simulink model "sampleModel256"  (R2021b)
settings: Solver=VariableStepAuto  StartTime=0.0  StopTime=10.0  RelTol=1e-3
undefined symbols (not defined in the file or in its folder): DiscIntNeverNeededParam
libraries: simulink x12, slpidlib x1
settings Model: Creator=user  LastModifiedBy=user

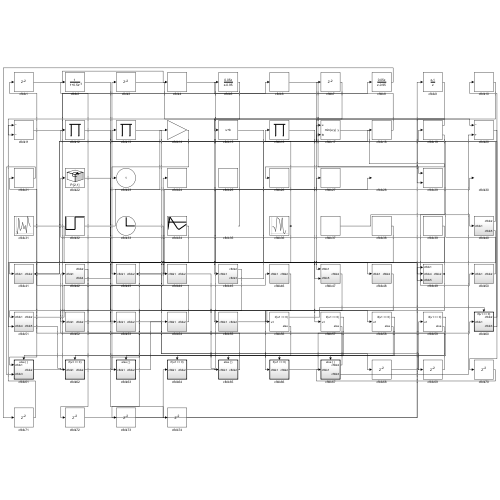
[thumbnail: Simulink's stored preview of the top-level diagram]
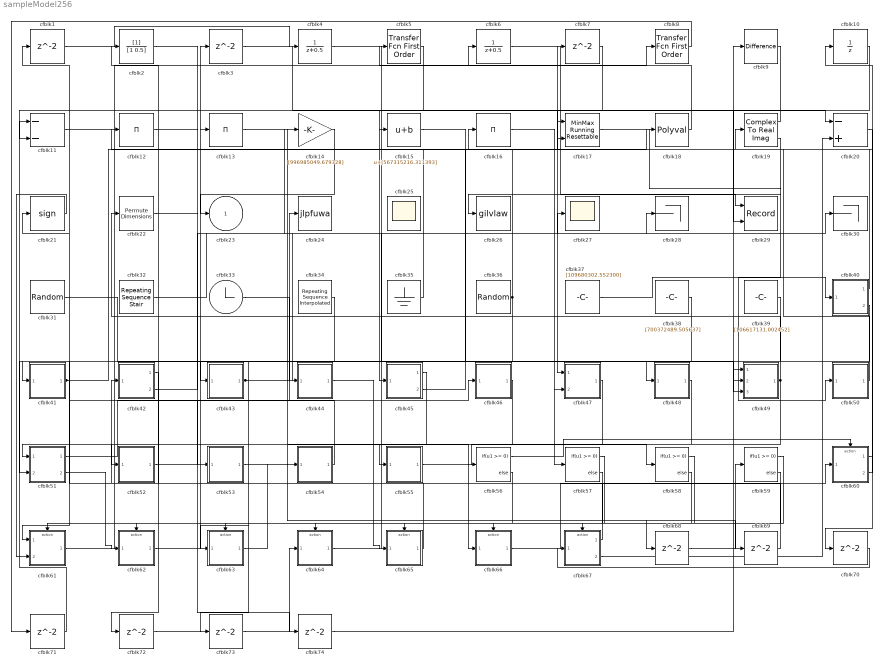
== system sampleModel256 ==
  cfblk{1,3,7,68..74} (10 alike) : Delay  SampleTime=1
  cfblk10 : UnitDelay  HasFrameUpgradeWarning=on
  cfblk11 : Sum  Inputs=--
  cfblk12 : Product  Inputs=*
  cfblk13 : Product  Inputs=*
  cfblk14 : Gain  Gain=[996985049.679328]
  cfblk15 : Bias  Bias=[567315216.311393]
  cfblk16 : Product  Inputs=*
  cfblk17 : simulink/Math Operations/MinMax Running Resettable  Function=min  vinit=0.0
  cfblk18 : Polyval  Coefs=[ +2.081618890e-019, -1.441693666e-014, +4.719686976e-010, -8.536869453e-006, +1.621573104e-001, -8.087801117e+001 ]
  cfblk19 : ComplexToRealImag
  cfblk2 : DiscreteFilter  SampleTime=1
  cfblk20 : Sum  Inputs=-+
  cfblk21 : Signum
  cfblk22 : PermuteDimensions
  cfblk24 : ToWorkspace  VariableName=jlpfuwa  SaveFormat=Timeseries  SampleTime=-1
  cfblk25 : Scope
      settings: Floating=on
  cfblk26 : ToWorkspace  VariableName=gilvlaw  SaveFormat=Timeseries  SampleTime=-1
  cfblk27 : Scope
  cfblk28 : Terminator
  cfblk29 : Record  FileSettingsInternal="{\"entries\":[{\"content\":{\"excelSettings\":{\"content\":{},\"type\":\"Streamout.ExcelSettings\"}},\"type\":\"Streamout.FileSettingStorage\",\"uuid\":\"d0f24451-51db-411e-8607-9f3c8963e8ef\"}],\"packageUris\":[\"http://schema.mathworks.com/mf0/streamout_blocks/R2020a\"],\"version\":\"1.0\"}"  Layout=[1 1]  SignalsInternal="{\"entries\":[{\"content\":{\"signals\":[{\"content\":{\"blockPath\":[\"sampleModel256/cfblk29\"],\"channel\":[],\"dimensions\":[1],\"domain\":\"sampleModel256/cfblk29\",\"lineColor\":\"#a2142f\",\"plots\":[1],\"port\":1,\"sid\":[\"\"],\"signalID\":10552,\"signalName\":\"cfblk6\"},\"type\":\"RecordBlkView.Signal\",\"uuid\":\"703fe235-f85b-4682-9098-29d6559715a6\"},{\"content\":{\"blockPath\":[\"sampleModel256/cfblk29\"],\"channel\":[],\"dimensions\":[1],\"domain\":\"sampleModel256/cfblk29\",\"lineColor\":\"#139fff\",\"plots\":[1],\"port\":2,\"sid\":[\"\"],\"signalID\":10556,\"signalName\":\"cfblk10\"},\"type\":\"RecordBlkView.Signal\",\"uuid\":\"3758a14b-5146-4c69-b112-1a56de22c7e5\"}]},\"type\":\"RecordBlkView.InputSignals\",\"uuid\":\"65a6738b-7d54-449a-83b2-f54919302c44\"}],\"packageUris\":[\"http://schema.mathworks.com/mf0/streamout_blocks/R2020a\"],\"version\":\"1.0\"}"  VisualizationBindings="{\"xyplotplugin\":{\"info\":[{\"series\":[{\"bindingParametersList\":[{\"parameter\":\"X-Axis\",\"signalID\":10552,\"signalName\":\"cfblk6\"},{\"parameter\":\"Y-Axis\",\"signalID\":10556,\"signalName\":\"cfblk10\"}],\"seriesID\":6340}],\"subplotID\":1}]}}"  CompatibilityTag=XY
  cfblk30 : Terminator
  cfblk31 : UniformRandomNumber  Minimum=[-810443101.783880]  Maximum=[9095802345.776228]  Seed=[48066271.000000]  SampleTime=0.1
  cfblk32 : simulink/Sources/Repeating Sequence Stair  OutValues=[667197621.575855, 764994376.330436]  tsamp=-1  OutMin=[]  OutMax=[]  OutDataTypeStr=double  OutputDataTypeScalingMode=double  OutDataType=fixdt(0,8)  ConRadixGroup=Best Precision: Vector-wise  OutScaling=2^-12
  cfblk33 : Clock
  cfblk34 : simulink/Sources/Repeating Sequence Interpolated  OutValues=[-652776122.372410, 660959935.276375, -741456881.763131, -889073054.086407, -257430787.269599]  TimeValues=[0 0.1 0.5 0.6 1].'  LookUpMeth=Interpolation-Use End Values  tsamp=0.01  OutMin=[]  OutMax=[]  OutDataTypeStr=double  OutputDataTypeScalingMode=double  OutDataType=fixdt(0,8)  OutScaling=2^-10
  cfblk35 : Ground
  cfblk36 : RandomNumber  Mean=[84976.409832]  Variance=[71029.152381]  Seed=[840926858.000000]  SampleTime=0.1
  cfblk37 : Constant  Value=[109680302.552300]  SampleTime=1
  cfblk38 : Constant  Value=[700372489.505637]  SampleTime=1
  cfblk39 : Constant  Value=[106617131.002452]  SampleTime=1
  cfblk4 : DiscreteTransferFcn  SampleTime=1
  cfblk40 : Subsystem
  cfblk41 : Subsystem
  cfblk42 : Subsystem
  cfblk43 : Subsystem
  cfblk44 : Subsystem
  cfblk45 : Subsystem
  cfblk46 : Subsystem
  cfblk47 : Subsystem
  cfblk48 : Subsystem
  cfblk49 : Subsystem
  cfblk5 : simulink/Discrete/Transfer Fcn First Order  PoleZ=0.95  ICPrevOutput=0.0  DoSatur=off
  cfblk50 : Subsystem
  cfblk51 : Subsystem
  cfblk52 : Subsystem
  cfblk53 : Subsystem
  cfblk54 : Subsystem
  cfblk55 : Subsystem
  cfblk{56..59} (4 alike) : If  IfExpression=u1 >= 0  SampleTime=1
  cfblk6 : DiscreteTransferFcn  SampleTime=1
  cfblk60 : Subsystem  TreatAsAtomicUnit=on
  cfblk61 : Subsystem  TreatAsAtomicUnit=on
  cfblk62 : Subsystem  TreatAsAtomicUnit=on
  cfblk63 : Subsystem  TreatAsAtomicUnit=on
  cfblk64 : Subsystem  TreatAsAtomicUnit=on
  cfblk65 : Subsystem  TreatAsAtomicUnit=on
  cfblk66 : Subsystem  TreatAsAtomicUnit=on
  cfblk67 : Subsystem  TreatAsAtomicUnit=on
  cfblk8 : simulink/Discrete/Transfer Fcn First Order  PoleZ=0.95  ICPrevOutput=0.0  DoSatur=off
  cfblk9 : simulink/Discrete/Difference  ICPrevInput=0.0  OutMin=[]  OutMax=[]  OutDataTypeStr=Inherit: Inherit via back propagation  OutDataType=fixdt(1, 16)  OutScaling=2^-10  DoSatur=off
  cfblk23 : Outport
  wires:
  cfblk3/1 -> cfblk20/1
  cfblk66/1(cfblk2) -> cfblk60/1(cfblk1)
  cfblk6/1 -> cfblk29/1
  cfblk51/1(cfblk2) -> cfblk24/1
  cfblk1/1 -> cfblk4/1
  cfblk32/1 -> cfblk14/1
  cfblk49/1(cfblk2) -> cfblk22/1, cfblk73/1
  cfblk7/1 -> cfblk47/1(cfblk1)
  cfblk60/1(cfblk2) -> cfblk10/1
  cfblk64/1(cfblk2) -> cfblk27/1
  cfblk47/1(cfblk2) -> cfblk55/1(cfblk1)
  cfblk16/1 -> cfblk57/1
  cfblk63/1(cfblk2) -> cfblk54/1(cfblk1)
  cfblk48/1(cfblk2) -> cfblk66/1(cfblk1)
  cfblk17/1 -> cfblk50/1(cfblk1)
  cfblk61/1(cfblk2) -> cfblk6/1
  cfblk38/1 -> cfblk41/1(cfblk1)
  cfblk4/1 -> cfblk48/1(cfblk1)
  cfblk44/1(cfblk2) -> cfblk65/1(cfblk1)
  cfblk62/1(cfblk2) -> cfblk3/1
  cfblk55/1(cfblk2) -> cfblk58/1
  cfblk18/1 -> cfblk5/1
  cfblk2/1 -> cfblk53/1(cfblk1)
  cfblk11/1 -> cfblk8/1
  cfblk37/1 -> cfblk40/1(cfblk1)
  cfblk35/1 -> cfblk12/1
  cfblk10/1 -> cfblk29/2
  cfblk60/2(cfblk3) -> cfblk13/1
  cfblk50/1(cfblk2) -> cfblk19/1
  cfblk52/1(cfblk2) -> cfblk46/1(cfblk1)
  cfblk9/1 -> cfblk45/1(cfblk1)
  cfblk43/1(cfblk2) -> cfblk30/1, cfblk56/1
  cfblk39/1 -> cfblk43/1(cfblk1)
  cfblk65/1(cfblk2) -> cfblk42/1(cfblk1)
  cfblk31/1 -> cfblk47/2(cfblk5)
  cfblk54/1(cfblk2) -> cfblk21/1
  cfblk19/1 -> cfblk15/1
  cfblk5/1 -> cfblk11/2
  cfblk14/1 -> cfblk23/1
  cfblk51/2(cfblk5) -> cfblk62/1(cfblk1)
  cfblk40/1(cfblk2) -> cfblk7/1
  cfblk33/1 -> cfblk44/1(cfblk1)
  cfblk36/1 -> cfblk16/1, cfblk51/2(cfblk4)
  cfblk19/2 -> cfblk26/1
  cfblk67/1(cfblk2) -> cfblk2/1
  cfblk41/1(cfblk2) -> cfblk18/1, cfblk17/2
  cfblk42/1(cfblk2) -> cfblk52/1(cfblk1)
  cfblk67/2(cfblk3) -> cfblk20/2
  cfblk15/1 -> cfblk49/2(cfblk4)
  cfblk40/2(cfblk5) -> cfblk63/1(cfblk1)
  cfblk45/1(cfblk2) -> cfblk51/1(cfblk1)
  cfblk12/1 -> cfblk49/3(cfblk5)
  cfblk42/2(cfblk4) -> cfblk28/1
  cfblk34/1 -> cfblk61/1(cfblk1)
  cfblk45/2(cfblk3) -> cfblk17/1
  cfblk21/1 -> cfblk61/2(cfblk3)
  cfblk56/1 -> cfblk60/Action
  cfblk56/2 -> cfblk61/Action
  cfblk57/1 -> cfblk62/Action
  cfblk57/2 -> cfblk63/Action
  cfblk58/1 -> cfblk64/Action
  cfblk58/2 -> cfblk65/Action
  cfblk59/1 -> cfblk66/Action
  cfblk59/2 -> cfblk67/Action
  cfblk13/1 -> cfblk68/1
  cfblk68/1 -> cfblk59/1
  cfblk53/1(cfblk2) -> cfblk69/1
  cfblk69/1 -> cfblk1/1
  cfblk20/1 -> cfblk70/1
  cfblk70/1 -> cfblk67/1(cfblk1)
  cfblk8/1 -> cfblk71/1
  cfblk71/1 -> cfblk11/1
  cfblk46/1(cfblk2) -> cfblk72/1
  cfblk72/1 -> cfblk64/1(cfblk1)
  cfblk73/1 -> cfblk9/1
  cfblk22/1 -> cfblk74/1
  cfblk74/1 -> cfblk49/1(cfblk1)

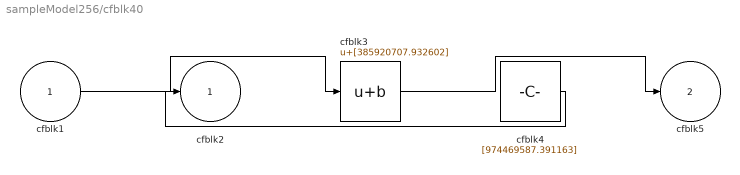
== system sampleModel256/cfblk40 ==
  cfblk1 : Inport
  cfblk3 : Bias  Bias=[385920707.932602]
  cfblk4 : Constant  Value=[974469587.391163]  SampleTime=1
  cfblk2 : Outport
  cfblk5 : Outport  Port=2
  wires:
  cfblk1/1 -> cfblk3/1
  cfblk4/1 -> cfblk2/1
  cfblk3/1 -> cfblk5/1

== system sampleModel256/cfblk41 ==
  cfblk1 : Inport
  cfblk3 : Sin  TimeSource=Use external signal  SampleTime=0
  cfblk2 : Outport
  wires:
  cfblk1/1 -> cfblk2/1, cfblk3/1

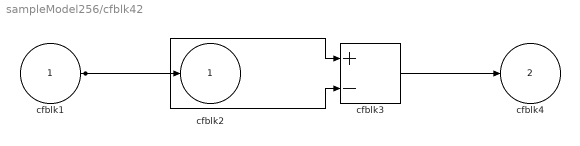
== system sampleModel256/cfblk42 ==
  cfblk1 : Inport
  cfblk3 : Sum  Inputs=+-
  cfblk2 : Outport
  cfblk4 : Outport  Port=2
  wires:
  cfblk1/1 -> cfblk3/1, cfblk3/2, cfblk2/1
  cfblk3/1 -> cfblk4/1

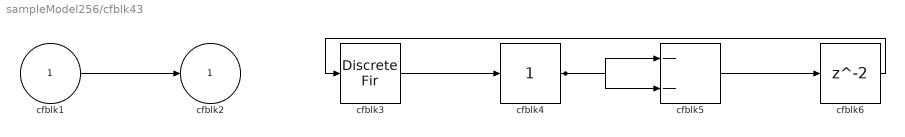
== system sampleModel256/cfblk43 ==
  cfblk1 : Inport
  cfblk3 : DiscreteFir  SampleTime=1
  cfblk4 : simulink/Math Operations/Slider Gain  gain=1  low=0  high=2
  cfblk5 : Sum  Inputs=--
  cfblk6 : Delay  SampleTime=1
  cfblk2 : Outport
  wires:
  cfblk3/1 -> cfblk4/1
  cfblk1/1 -> cfblk2/1
  cfblk4/1 -> cfblk5/1, cfblk5/2
  cfblk5/1 -> cfblk6/1
  cfblk6/1 -> cfblk3/1

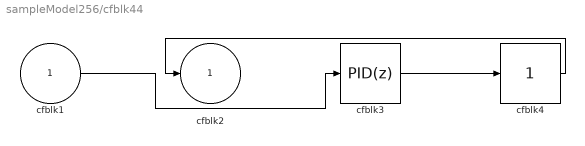
== system sampleModel256/cfblk44 ==
  cfblk1 : Inport
  cfblk3 : slpidlib/PID Controller  Controller=PID  Form=Parallel  TimeDomain=Discrete-time  UseExternalTs=off  SampleTime=1  IntegratorMethod=Forward Euler  FilterMethod=Forward Euler  ControllerParametersSource=internal  P=1  I=1  D=0  UseFilter=on  N=100  TunerSelectOption=Transfer Function Based (PID Tuner App)  InitialConditionSource=internal  InitialConditionForIntegrator=0  InitialConditionForFilter=0  DifferentiatorICPrevScaledInput=0  ExternalReset=none  TrackingMode=off  Kt=1  LimitOutput=off  SatLimitsSource=internal  UpperSaturationLimit=inf  LowerSaturationLimit=-inf  LinearizeAsGain=off  AntiWindupMode=none  Kb=1  POutMin=[]  POutMax=[]  IOutMin=[]  IOutMax=[]  DOutMin=[]  DOutMax=[]  NOutMin=[]  NOutMax=[]  SumOutMin=[]  SumOutMax=[]  SaturationOutMin=[]  SaturationOutMax=[]  PParamMin=[]  PParamMax=[]  IParamMin=[]  IParamMax=[]  DParamMin=[]  DParamMax=[]  NParamMin=[]  NParamMax=[]  KbParamMin=[]  KbParamMax=[]  KtParamMin=[]  KtParamMax=[]  KbOutMin=[]  KbOutMax=[]  KtOutMin=[]  KtOutMax=[]  IntegratorOutMin=[]  IntegratorOutMax=[]  FilterOutMin=[]  FilterOutMax=[]  SumI1OutMin=[]  SumI1OutMax=[]  SumI2OutMin=[]  SumI2OutMax=[]  SumI3OutMin=[]  SumI3OutMax=[]  SumI4OutMin=[]  SumI4OutMax=[]  SumDOutMin=[]  SumDOutMax=[]  DifferentiatorOutMin=[]  DifferentiatorOutMax=[]  FilterDiffOutCoefMin=[]  FilterDiffOutCoefMax=[]  ReciprocalOutMin=[]  ReciprocalOutMax=[]  SumDenOutMin=[]  SumDenOutMax=[]  SumNumOutMin=[]  SumNumOutMax=[]  DivideOutMin=[]  DivideOutMax=[]  UdiffTsProdOutMin=[]  UdiffTsProdOutMax=[]  NTsProdOutMin=[]  NTsProdOutMax=[]  UintegralTsProdOutMin=[]  UintegralTsProdOutMax=[]  UngainTsProdOutMin=[]  UngainTsProdOutMax=[]  IntegratorContinuousStateAttributes=''  IntegratorStateMustResolveToSignalObject=off  IntegratorRTWStateStorageClass=Auto  FilterContinuousStateAttributes=''  FilterStateMustResolveToSignalObject=off  FilterRTWStateStorageClass=Auto  ParallelPVariant=InternalParameters  IdealPVariant=Disabled  IVariant=InternalParameters  DVariant=InternalParameters  IntegratorVariant=Discrete  SatVariant=Disabled  AWVariant=Passthrough  PCopyVariant=Disabled  TRVariant=Disabled  FdbkBlocksVariant=Forward  IdealPFdbkVariant=Disabled  SatFdbkVariant=Disabled  DerivativeFilterVariant=ForwardEulerFilter  NVariant=InternalParameters  NCopyVariant=Disabled  FilterICVariant=InternalICsFilter  IntegratorICVariant=InternalICs  ExternalResetVariant=Disabled  TRSumVariant=Passthrough  SumFdbkVariant=Disabled  SumVariant=Sum_PID  TsampFilterVariant=InternalTs  TsampNgainVariant=Passthrough  TsampIntegralVariant=Passthrough  ExternalSaturationOutDataTypeStr=Inherit: Same as second input
  cfblk4 : simulink/Math Operations/Slider Gain  gain=1  low=0  high=2
  cfblk2 : Outport
  wires:
  cfblk3/1 -> cfblk4/1
  cfblk4/1 -> cfblk2/1
  cfblk1/1 -> cfblk3/1

== system sampleModel256/cfblk45 ==
  cfblk1 : Inport
  cfblk2 : Outport
  cfblk3 : Outport  Port=2
  wires:
  cfblk1/1 -> cfblk3/1, cfblk2/1

== system sampleModel256/cfblk46 ==
  cfblk1 : Inport
  cfblk3 : DiscreteStateSpace
  cfblk2 : Outport
  wires:
  cfblk1/1 -> cfblk3/1
  cfblk3/1 -> cfblk2/1

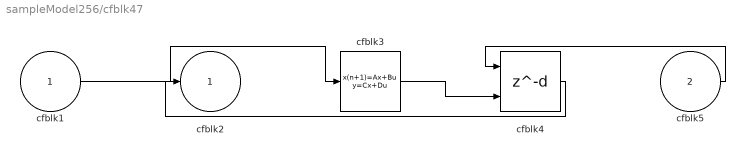
== system sampleModel256/cfblk47 ==
  cfblk1 : Inport
  cfblk5 : Inport  Port=2
  cfblk3 : DiscreteStateSpace
  cfblk4 : Delay  DelayLengthSource=Input port  SampleTime=1
      settings: InputPortMap=u0,p1
  cfblk2 : Outport
  wires:
  cfblk1/1 -> cfblk3/1
  cfblk5/1 -> cfblk4/1
  cfblk3/1 -> cfblk4/2
  cfblk4/1 -> cfblk2/1

== system sampleModel256/cfblk48 ==
  cfblk1 : Inport
  cfblk3 : DiscreteIntegrator  ICPrevOutput=DiscIntNeverNeededParam  ICPrevScaledInput=DiscIntNeverNeededParam
  cfblk2 : Outport
  wires:
  cfblk1/1 -> cfblk3/1
  cfblk3/1 -> cfblk2/1

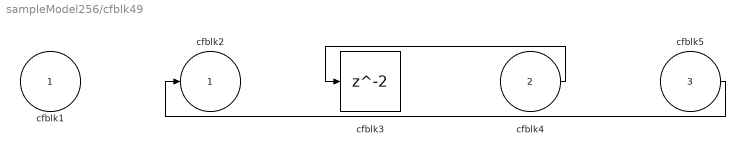
== system sampleModel256/cfblk49 ==
  cfblk1 : Inport
  cfblk4 : Inport  Port=2
  cfblk5 : Inport  Port=3
  cfblk3 : Delay  SampleTime=1
  cfblk2 : Outport
  wires:
  cfblk4/1 -> cfblk3/1
  cfblk5/1 -> cfblk2/1

== system sampleModel256/cfblk50 ==
  cfblk1 : Inport
  cfblk3 : DiscreteFir  SampleTime=1
  cfblk2 : Outport
  wires:
  cfblk1/1 -> cfblk3/1
  cfblk3/1 -> cfblk2/1

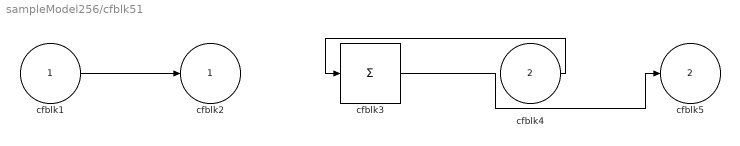
== system sampleModel256/cfblk51 ==
  cfblk1 : Inport
  cfblk4 : Inport  Port=2
  cfblk3 : Sum  Inputs=+
  cfblk2 : Outport
  cfblk5 : Outport  Port=2
  wires:
  cfblk1/1 -> cfblk2/1
  cfblk4/1 -> cfblk3/1
  cfblk3/1 -> cfblk5/1

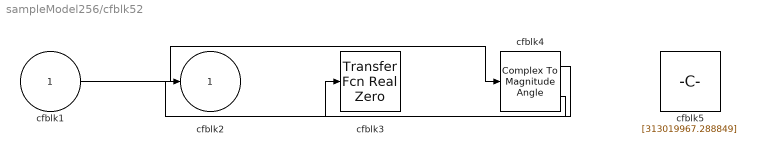
== system sampleModel256/cfblk52 ==
  cfblk1 : Inport
  cfblk3 : simulink/Discrete/Transfer Fcn Real Zero  ZeroZ=0.75  ICPrevInput=0.0  DoSatur=off
      settings: SourceProductBaseCode=SL
  cfblk4 : ComplexToMagnitudeAngle
  cfblk5 : Constant  Value=[313019967.288849]  SampleTime=1
  cfblk2 : Outport
  wires:
  cfblk1/1 -> cfblk4/1
  cfblk4/1 -> cfblk3/1
  cfblk4/2 -> cfblk2/1

== system sampleModel256/cfblk53 ==
  cfblk1 : Inport
  cfblk3 : Delay  ShowEnablePort=on  SampleTime=1
      settings: InputPortMap=u0,e6
  cfblk2 : Outport
  wires:
  cfblk1/1 -> cfblk3/1, cfblk3/2
  cfblk3/1 -> cfblk2/1

== system sampleModel256/cfblk54 ==
  cfblk1 : Inport
  cfblk3 : simulink/Math Operations/MinMax Running Resettable  Function=min  vinit=0.0
  cfblk2 : Outport
  wires:
  cfblk1/1 -> cfblk3/1, cfblk3/2
  cfblk3/1 -> cfblk2/1

== system sampleModel256/cfblk55 ==
  cfblk1 : Inport
  cfblk3 : Sum  Inputs=+-
  cfblk2 : Outport
  wires:
  cfblk1/1 -> cfblk2/1, cfblk3/1, cfblk3/2

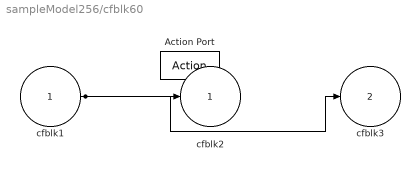
== system sampleModel256/cfblk60 ==
  cfblk1 : Inport
  Action Port : ActionPort  ActionPortLabel=if(u1 >= 0)
  cfblk2 : Outport
  cfblk3 : Outport  Port=2
  wires:
  cfblk1/1 -> cfblk3/1, cfblk2/1

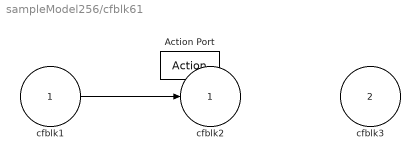
== system sampleModel256/cfblk61 ==
  cfblk1 : Inport
  cfblk3 : Inport  Port=2
  Action Port : ActionPort  ActionPortLabel=else
  cfblk2 : Outport
  wires:
  cfblk1/1 -> cfblk2/1

== system sampleModel256/cfblk62 ==
  cfblk1 : Inport
  Action Port : ActionPort  ActionPortLabel=if(u1 >= 0)
  cfblk3 : Sum  Inputs=|++
  cfblk2 : Outport
  wires:
  cfblk1/1 -> cfblk3/1, cfblk3/2
  cfblk3/1 -> cfblk2/1

== system sampleModel256/cfblk63 ==
  cfblk1 : Inport
  Action Port : ActionPort  ActionPortLabel=else
  cfblk3 : Bias  Bias=[432812070.396524]
  cfblk2 : Outport
  wires:
  cfblk1/1 -> cfblk3/1
  cfblk3/1 -> cfblk2/1

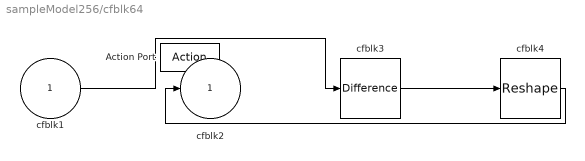
== system sampleModel256/cfblk64 ==
  cfblk1 : Inport
  Action Port : ActionPort  ActionPortLabel=if(u1 >= 0)
  cfblk3 : simulink/Discrete/Difference  ICPrevInput=0.0  OutMin=[]  OutMax=[]  OutDataTypeStr=Inherit: Inherit via back propagation  OutDataType=fixdt(1, 16)  OutScaling=2^-10  DoSatur=off
  cfblk4 : Reshape
  cfblk2 : Outport
  wires:
  cfblk4/1 -> cfblk2/1
  cfblk3/1 -> cfblk4/1
  cfblk1/1 -> cfblk3/1

== system sampleModel256/cfblk65 ==
  cfblk1 : Inport
  Action Port : ActionPort  ActionPortLabel=else
  cfblk3 : simulink/Math Operations/MinMax Running Resettable  Function=min  vinit=0.0
  cfblk2 : Outport
  wires:
  cfblk1/1 -> cfblk3/1, cfblk3/2
  cfblk3/1 -> cfblk2/1

== system sampleModel256/cfblk66 ==
  cfblk1 : Inport
  Action Port : ActionPort  ActionPortLabel=if(u1 >= 0)
  cfblk3 : UnaryMinus
  cfblk2 : Outport
  wires:
  cfblk3/1 -> cfblk2/1
  cfblk1/1 -> cfblk3/1

== system sampleModel256/cfblk67 ==
  cfblk1 : Inport
  Action Port : ActionPort  ActionPortLabel=else
  cfblk2 : Outport
  cfblk3 : Outport  Port=2
  wires:
  cfblk1/1 -> cfblk2/1, cfblk3/1
